simulink model "SG__MDL"  (R2022b)
settings: Solver=FixedStepAuto  StartTime=0.0  StopTime=Inf  FixedStep=5e-05  RelTol=1e-3  EnableMultiTasking=on
model workspace (MAT data in the model file):
  N_trig = Simulink.Parameter
  N_trig.Value = 32
  N_trig.Description = 'number of samples for triggered pulse for recording'
  N_trig.DataType = 'uint32'
  N_trig.Complexity = 'real'
  N_trig.Dimensions = [1 1]
  Sig = Simulink.Signal
  Sig.DataType = 'auto'
  Sig.Dimensions = -1
  Sig.DimensionsMode = 'auto'
  Sig.Complexity = 'auto'
  Sig.SampleTime = -1
  Sig.SamplingMode = 'auto'
  dtf_a = Simulink.Parameter
  dtf_a.Value = [1  1  1; 1  1  1]
  dtf_a.DataType = 'auto'
  dtf_a.Complexity = 'real'
  dtf_a.Dimensions = [2 3]
  dtf_b = Simulink.Parameter
  dtf_b.Value = [0.5  0.5  0.5; 0.5  0.5  0.5]
  dtf_b.DataType = 'auto'
  dtf_b.Complexity = 'real'
  dtf_b.Dimensions = [2 3]
  freq_0 = Simulink.Parameter
  freq_0.Value = 602
  freq_0.Description = 'tube fundamental resonance frequency
    | '
  freq_0.DataType = 'auto'
  freq_0.Complexity = 'real'
  freq_0.Dimensions = [1 1]
  i2u = Simulink.Parameter
  i2u.Value = 100
  i2u.Description = 'current to voltage conversion'
  i2u.DataType = 'auto'
  i2u.Complexity = 'real'
  i2u.Dimensions = [1 1]
  phi = Simulink.Parameter
  phi.Value = [0; 0]
  phi.DataType = 'auto'
  phi.Complexity = 'real'
  phi.Dimensions = [2 1]
  rec = Simulink.Parameter
  rec.Value = 0
  rec.DataType = 'boolean'
  rec.Complexity = 'real'
  rec.Dimensions = [1 1]
  rho = Simulink.Parameter
  rho.Value = [1; 1]
  rho.DataType = 'auto'
  rho.Complexity = 'real'
  rho.Dimensions = [2 1]
  sens_p = Simulink.Parameter
  sens_p.Value = [0; 0]
  sens_p.DataType = 'auto'
  sens_p.Complexity = 'real'
  sens_p.Dimensions = [2 1]
  src_gain = Simulink.Parameter
  src_gain.Value = 0.05
  src_gain.DataType = 'auto'
  src_gain.Complexity = 'real'
  src_gain.Dimensions = [1 1]
  theta = Simulink.Parameter
  theta.Value = [3.14159265359; 0]
  theta.DataType = 'auto'
  theta.Complexity = 'real'
  theta.Dimensions = [2 1]
  ts_ctr = Simulink.Parameter
  ts_ctr.Value = 5e-05
  ts_ctr.DataType = 'auto'
  ts_ctr.Complexity = 'real'
  ts_ctr.Dimensions = [1 1]
undefined symbols (not defined in the file or in its folder): gcbh, sps, sps_rtmsupport, t_s
libraries: simulink x3, speedgoatlib_IO135 x3, spsMeanLib x2, hdlsllib x2, slrealtimeloglib x1, dspsigops x1
settings Model: SimulationMode=external  ExtModeEnableFloating=off  DataflowThreadingImplementation=Pthreads  Creator=padlewsk  LastModifiedBy=padlewsk
settings SolverCC: ConcurrentTasks=on  AlgebraicLoopSolver=TrustRegion  PositivePriorityOrder=on  AutoInsertRateTranBlk=on
settings DataIOCC: SaveFormat=StructureWithTime
settings OptimizationCC: DefaultParameterBehavior=Inlined  GainParamInheritBuiltInType=on  UseFloatMulNetSlope=on  RollThreshold=9  EfficientFloat2IntCast=on  SimCompilerOptimization=on
settings DebuggingCC: ReadBeforeWriteMsg=DisableAll  WriteAfterWriteMsg=DisableAll  WriteAfterReadMsg=DisableAll  TasksWithSamePriorityMsg=none  UnconnectedInputMsg=warning  UnconnectedOutputMsg=warning  UnconnectedLineMsg=warning  ModelReferenceSymbolNameMessage=none
settings HardwareCC: ProdBitPerLong=64  ProdLongLongMode=on  ProdHWDeviceType=Intel->x86-64 (Linux 64)
settings ModelReferenceCC: UpdateModelReferenceTargets=IfOutOfDate  EnableRefExpFcnMdlSchedulingChecks=on
settings SFSimCC: SFSimEcho=off
settings RTWCC: Description=Simulink Real-Time  SystemTargetFile=slrealtime.tlc  TemplateMakefile=slrealtime_default_tmf  Toolchain=Simulink Real-Time Toolchain  BuildConfiguration=Faster Runs  CodeExecutionProfiling=on  TargetLang=C++
settings SimulinkRealTimeTargetCC: UseGCCFastMath=on

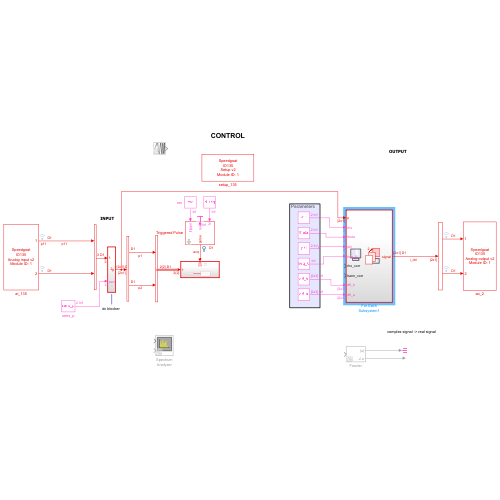
[thumbnail: Simulink's stored preview of the top-level diagram]
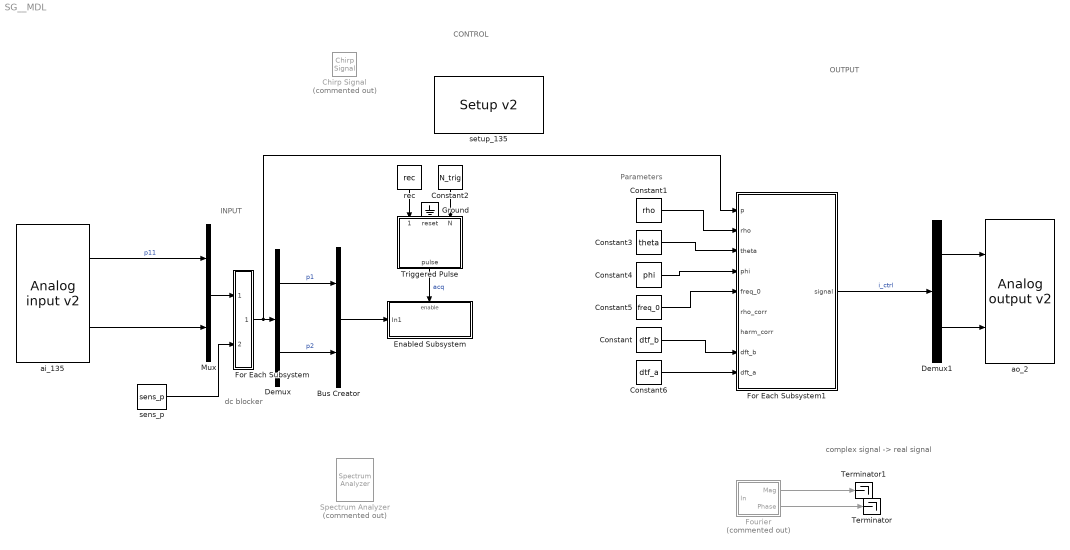
== system SG__MDL ==
  note: complex signal -> real signal
  note: dc blocker
  note: OUTPUT
  note: Parameters
  note: CONTROL
  note: INPUT
  Bus Creator : BusCreator  Inputs=2
  Chirp Signal : simulink/Sources/Chirp Signal  Commented=on  f1=10  T=10  f2=1500
  Constant : Constant  Value=dtf_b
  Constant1 : Constant  Value=rho
  Constant2 : Constant  Value=N_trig
  Constant3 : Constant  Value=theta
  Constant4 : Constant  Value=phi
  Constant5 : Constant  Value=freq_0
  Constant6 : Constant  Value=dtf_a
  Demux : Demux  Outputs=2
  Demux1 : Demux  Outputs=2
  Enabled Subsystem : Subsystem  TreatAsAtomicUnit=on
  For Each Subsystem : Subsystem  TreatAsAtomicUnit=on
  For Each Subsystem1 : Subsystem  TreatAsAtomicUnit=on
  Fourier : Subsystem  Commented=on  DialogController=POWERSYS.PowerSysDialog  LoadFcn=sps_rtmsupport('LoadFcn', gcbh);  StartFcn=sps_rtmsupport('StartFcn', gcbh);  StopFcn=sps_rtmsupport('StopFcn', gcbh);  mask(Fourier){Freq=freq_0, n=0, InInit=[0, 0], Ts=t_s}
      mask prompts: Freq "Fundamental frequency (Hz):"; n "Harmonic n (0=DC, 1=fundamental):"; InInit "Initial input [ Mag, Phase (degrees) ]:"; Ts "Sample time:"
      mask help:
      | Fourier analysis of the input signal over a running window of one cycle of the fundamental frequency.
      |
      | For the first cycle of simulation, the outputs are held  to the value specified in the Initial input parameter.
      mask init:
      | [WantBlockChoice,Ts,sps] = powericon('FourierInit',gcb,Freq,n,InInit,Ts);
      settings: LibrarySourceBlock=sps_lib/Sensors and Measurements/Fourier  CopyFcn=sps_rtmsupport('CopyFcn', gcbh);  DeleteFcn=sps_rtmsupport('DeleteFcn', gcbh);  UndoDeleteFcn=sps_rtmsupport('UndoDeleteFcn', gcbh);  ModelCloseFcn=sps_rtmsupport('ModelCloseFcn', gcbh);  PreSaveFcn=sps_rtmsupport('PreSaveFcn', gcbh);  PostSaveFcn=sps_rtmsupport('PostSaveFcn', gcbh);  NameChangeFcn=sps_rtmsupport('NameChangeFcn', gcbh);  PreCopyFcn=sps_rtmsupport('PreCopyFcn', gcbh);  OpenFcn=sps_rtmsupport('OpenFcn', gcbh, []);  CloseFcn=sps_rtmsupport('CloseFcn', gcbh);  PreDeleteFcn=sps_rtmsupport('PreDeleteFcn', gcbh);
      mask Help: helpview(psbhelp);
      mask Display:
      | port_label('output',1,'|u|')
      | port_label('output',2,'\angleu', 'texmode', 'on')
  Ground : Ground
  Mux : Mux  Inputs=2
  Spectrum Analyzer : SpectrumAnalyzer  Commented=on  NumInputPorts=2
  Terminator : Terminator
  Terminator1 : Terminator
  Triggered Pulse : Subsystem  mask(Triggered Pulse){}
      mask help: Generates a single pulse of N samples length
  ai_135 : speedgoatlib_IO135/Analog input v2   parModuleId=1  parSampleTime=-1  parPciSlot=-1  parAdcChannels=[1 2]  parAdcVoltageRange=[1 1 1 1]  parAdcOversamplRate=[1 1 1 1]  parAdcContSampling=0  parAdcDmaEnable=0  parAdcActiveDmaDevices=[1 1 1 1]  parAdcFrameSize=1
      settings: SourceProductName=Simulink Real-Time: Speedgoat I/O Blockset
  ao_2 : speedgoatlib_IO135/Analog output v2   parModuleId=1  parSampleTime=-1  parPciSlot=-1  parDacChannels=[1 2]  parDacVoltageRange=[4 4 4 4 4 4 4 4 4 4 4 4 4 4 4 4]  parDacInitValues=[0 0]  parDacReset=[1 1]  parDacSyncOut=1  parDacDmaEnable=0  parDacActiveDmaDevices=[1 1 1 1]  parDacDmaLatency=1  parDacFrameSize=1
      settings: SourceProductName=Simulink Real-Time: Speedgoat I/O Blockset
  rec : Constant  Value=rec
  sens_p : Constant  Value=sens_p
  setup_135 : speedgoatlib_IO135/Setup v2   parPciSlot=-1  parModuleId=1  parInterModuleSync=None  parConvClockBaseRate=20MHz  parConvClock1Divider=700  parConvClock2Divider=700  parFrameTriggerEnable=off  parFrameTriggerDivider=10  parConvClock1BaseRate=1  parConvClock2BaseRate=1  parFrameTriggerClock=1  parAdcChannels=[1:2]  parAdcRange1=+-5V  parAdcRange2=+-5V  parAdcRange3=+-5V  parAdcRange4=+-5V  parAdcVoltageRange=[1 1 1 1]  parAdcOversampling1=None  parAdcOversampling2=None  parAdcOversampling3=None  parAdcOversampling4=None  parAdcOversamplRate=[1 1 1 1]  parAdcAutoCorrection=on  parAdcContSampling=off  parAdcDmaEnable=off  parAdcDmaClock=Clock 1  parAdcFrameSize_=1  parAdcSampleTime_=-1  parAdcActiveDmaDevices=[1 1 1 1]  parAdcFrameTriggerEnable=0  parAdcFrameSize=1  parAdcSampleTime=3.5e-05  parDacChannels=[1:2]  parDacInitValues=zeros(1,2)  parDacReset=1  parDacRange1=+-5V  parDacRange2=+-5V  parDacRange3=+-5V  parDacRange4=+-5V  parDacRange5=+-5V  parDacRange6=+-5V  parDacRange7=+-5V  parDacRange8=+-5V  parDacRange9=+-5V  parDacRange10=+-5V  parDacRange11=+-5V  parDacRange12=+-5V  parDacRange13=+-5V  parDacRange14=+-5V  parDacRange15=+-5V  parDacRange16=+-5V  parDacVoltageRange=[4 4 4 4 4 4 4 4 4 4 4 4 4 4 4 4]  parDacAutoCorrection=on  parDacSyncOut=on  parDacDmaEnable=off  parDacDmaLatency=As small as possible  parDacDmaClock=Clock 1  parDacFrameSize_=1  parDacSampleTime_=-1  parDacActiveDmaDevices=[1 1 1 1]  parDacFrameTriggerEnable=0  parDacFrameSize=1  parDacSampleTime=3.5e-05  parDoChannels=[]  parDoInitValues=0  parDoReset=1  parDiChannels=[]  parDiDebounceEnable=off  parDiDebounceTime=0  parDiDebounceValue=0  parDioPullRefFront=Pull-up 3.3V  parDioPullRefRear=Floating
      settings: SourceProductName=Simulink Real-Time: Speedgoat I/O Blockset
  wires:
  ai_135/2 -> Mux/2
  ai_135/1 -> Mux/1  "p11"
  Mux/1 -> For Each Subsystem/1(In1)
  For Each Subsystem/1(p) -> For Each Subsystem1/1(p), Demux/1
  Bus Creator/1 -> Enabled Subsystem/1(In1)
  Demux/1 -> Bus Creator/1  "p1"
  Demux/2 -> Bus Creator/2  "p2"
  Triggered Pulse/1(pulse) -> Enabled Subsystem/Enable  "acq"
  Ground/1 -> Triggered Pulse/2(reset)
  rec/1 -> Triggered Pulse/1(trigger)
  Constant2/1 -> Triggered Pulse/3(N)
  Constant1/1 -> For Each Subsystem1/2(rho)
  Constant3/1 -> For Each Subsystem1/3(theta)
  Constant4/1 -> For Each Subsystem1/4(phi)
  Constant5/1 -> For Each Subsystem1/5(freq_0)
  Demux1/1 -> ao_2/1
  Demux1/2 -> ao_2/2
  Fourier/2(Phase) -> Terminator/1
  Fourier/1(Mag) -> Terminator1/1
  Constant6/1 -> For Each Subsystem1/9(dft_a)
  Constant/1 -> For Each Subsystem1/8(dft_b)
  For Each Subsystem1/1(signal) -> Demux1/1  "i_ctrl"
  sens_p/1 -> For Each Subsystem/2(sens_p)

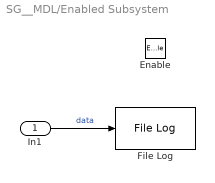
== system SG__MDL/Enabled Subsystem ==
  In1 : Inport
  Enable : EnablePort
  File Log : slrealtimeloglib/File Log  decimation=1  inputProcessing=Elements as channels (sample based)
  wires:
  In1/1 -> File Log/1  "data"

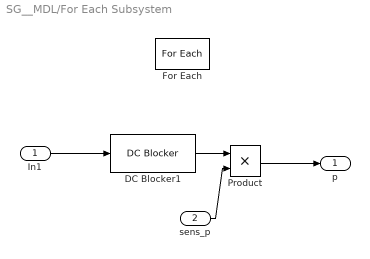
== system SG__MDL/For Each Subsystem ==
  In1 : Inport  Partition=on  PartitionDimension=1  PartitionWidth=1  PartitionOffset=0
  sens_p : Inport  Port=2  Partition=on  PartitionDimension=1  PartitionWidth=1  PartitionOffset=0
  DC Blocker1 : dspsigops/DC Blocker  Algorithm=IIR  NormalizedBandwidth=0.001  Length=50  Order=3  SimulateUsing=Code generation
      settings: LibrarySourceBlock=dsphdlsupportsigops/DC Blocker
  For Each : ForEach  DisableCoverage=on
  Product : Product
  p : Outport  ConcatenationDimension=1
  wires:
  In1/1 -> DC Blocker1/1
  DC Blocker1/1 -> Product/1
  Product/1 -> p/1
  sens_p/1 -> Product/2

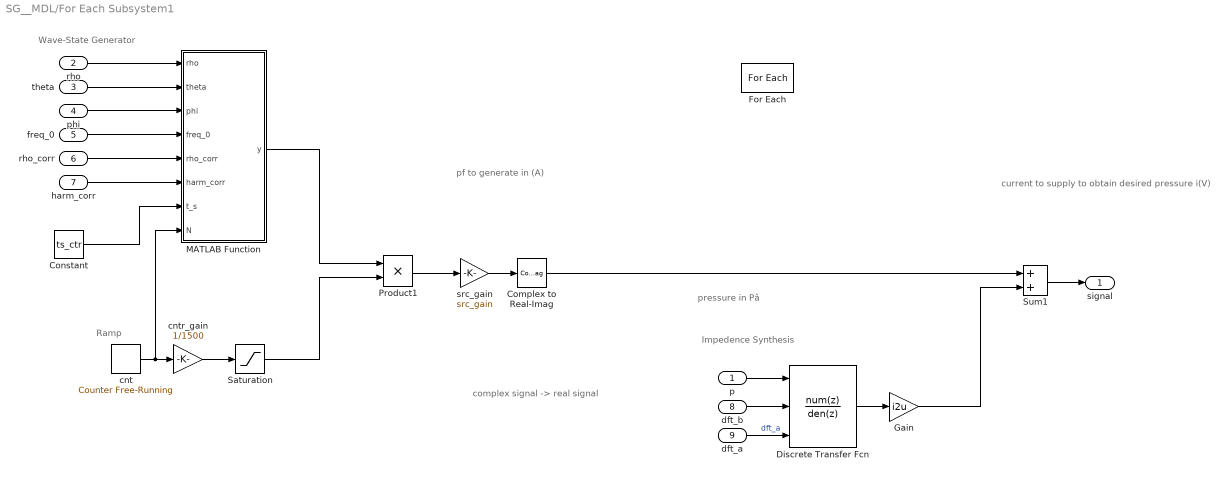
== system SG__MDL/For Each Subsystem1 ==
  note: pressure in Pâ
  note: pf to generate in (A)
  note: Wave-State Generator
  note: Impedence Synthesis
  note: Ramp
  note: complex signal -> real signal
  note: current to supply to obtain desired pressure i(V)
  p : Inport  Partition=on  PartitionDimension=1  PartitionWidth=1  PartitionOffset=0
  rho : Inport  Port=2  Partition=on  PartitionDimension=1  PartitionWidth=1  PartitionOffset=0
  theta : Inport  Port=3  Partition=on  PartitionDimension=1  PartitionWidth=1  PartitionOffset=0
  phi : Inport  Port=4  Partition=on  PartitionDimension=1  PartitionWidth=1  PartitionOffset=0
  freq_0 : Inport  Port=5
  rho_corr : Inport  Port=6
  harm_corr : Inport  Port=7
  dft_b : Inport  Port=8  Partition=on  PartitionDimension=1  PartitionWidth=1  PartitionOffset=0
  dft_a : Inport  Port=9  Partition=on  PartitionDimension=1  PartitionWidth=1  PartitionOffset=0
  Complex to Real-Imag : ComplexToRealImag  Output=Real
  Constant : Constant  Value=ts_ctr  SampleTime=-1
  Discrete Transfer Fcn : DiscreteTransferFcn  NumeratorSource=Input port  DenominatorSource=Input port  a0EqualsOne=on
      settings: InputPortMap=u0,p1,p3
  For Each : ForEach  DisableCoverage=on
  Gain : Gain  Gain=i2u
  MATLAB Function : MATLAB Function  TreatAsAtomicUnit=on
  Product1 : Product
  Saturation : Saturate  UpperLimit=1  LowerLimit=0
  Sum1 : Sum
  cnt : simulink/Sources/Counter Free-Running  NumBits=32  tsamp=-1
  cntr_gain : Gain  Gain=1/1500  ParamDataTypeStr=double
  src_gain : Gain  Gain=src_gain
  signal : Outport  OutputWhenDisabled=reset  InitialOutput=0  ConcatenationDimension=1  VectorParamsAs1DForOutWhenUnconnected=off
  wires:
  freq_0/1 -> MATLAB Function/4(freq_0)
  rho/1 -> MATLAB Function/1(rho)
  cnt/1 -> MATLAB Function/8(N), cntr_gain/1
  Product1/1 -> src_gain/1
  phi/1 -> MATLAB Function/3(phi)
  theta/1 -> MATLAB Function/2(theta)
  Saturation/1 -> Product1/2
  cntr_gain/1 -> Saturation/1
  Constant/1 -> MATLAB Function/7(t_s)
  MATLAB Function/1(y) -> Product1/1
  dft_b/1 -> Discrete Transfer Fcn/2
  dft_a/1 -> Discrete Transfer Fcn/3  "dft_a"
  src_gain/1 -> Complex to Real-Imag/1
  Discrete Transfer Fcn/1 -> Gain/1
  Gain/1 -> Sum1/2
  Sum1/1 -> signal/1
  p/1 -> Discrete Transfer Fcn/1
  Complex to Real-Imag/1 -> Sum1/1
  rho_corr/1 -> MATLAB Function/5(rho_corr)
  harm_corr/1 -> MATLAB Function/6(harm_corr)

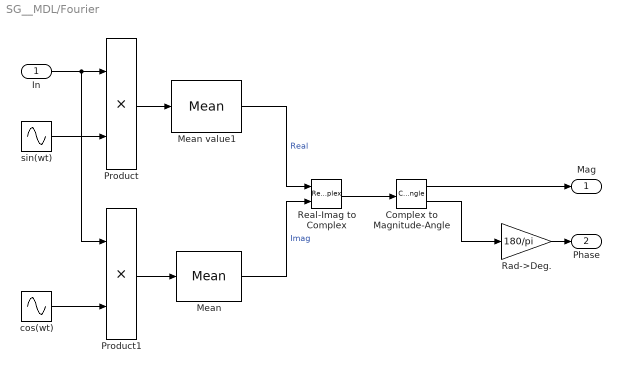
== system SG__MDL/Fourier ==
  In : Inport  SampleTime=Ts
  Complex to Magnitude-Angle : ComplexToMagnitudeAngle
  Mean : spsMeanLib/Mean  Freq=sps.Freq  Vinit=sps.Imag_Init  Ts=Ts
  Mean value1 : spsMeanLib/Mean  Freq=sps.Freq  Vinit=sps.Real_Init  Ts=Ts
  Product : Product  InputSameDT=on  SaturateOnIntegerOverflow=on  OutDataTypeStr=Inherit: Same as first input
  Product1 : Product  InputSameDT=on  SaturateOnIntegerOverflow=on  OutDataTypeStr=Inherit: Same as first input
  Rad->Deg. : Gain  Gain=180/pi  SaturateOnIntegerOverflow=on  OutDataTypeStr=Inherit: Same as input  ParamDataTypeStr=Inherit: Same as input
  Real-Imag to Complex : RealImagToComplex
  cos(wt) : Sin  Amplitude=sps.k  Frequency=2*pi*Freq*sps.n  Phase=pi/2  SampleTime=Ts
  sin(wt) : Sin  Amplitude=sps.k  Frequency=2*pi*Freq*sps.n  SampleTime=Ts
  Mag : Outport  SampleTime=Ts  VectorParamsAs1DForOutWhenUnconnected=off
  Phase : Outport  Port=2  SampleTime=Ts  VectorParamsAs1DForOutWhenUnconnected=off
  wires:
  In/1 -> Product/1, Product1/1
  sin(wt)/1 -> Product/2
  Product/1 -> Mean value1/1
  Mean value1/1 -> Real-Imag to Complex/1  "Real"
  Mean/1 -> Real-Imag to Complex/2  "Imag"
  Complex to Magnitude-Angle/1 -> Mag/1
  Rad->Deg./1 -> Phase/1
  Real-Imag to Complex/1 -> Complex to Magnitude-Angle/1
  Complex to Magnitude-Angle/2 -> Rad->Deg./1
  cos(wt)/1 -> Product1/2
  Product1/1 -> Mean/1

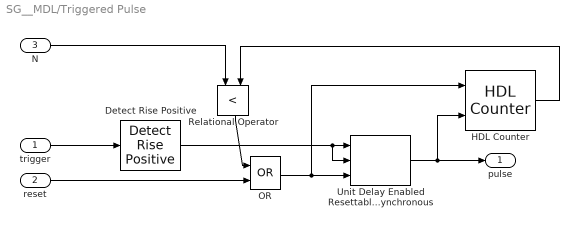
== system SG__MDL/Triggered Pulse ==
  trigger : Inport
  reset : Inport  Port=2
  N : Inport  Port=3
  Detect Rise Positive : simulink/Logic and Bit Operations/Detect Rise Positive  vinit=0  OutDataTypeStr=boolean
  HDL Counter : hdlsllib/Sources/HDL Counter  CountType=Free running  CountInit=1  CountStep=1  CountMax=25  CountFromType=Initial value  CountFrom=1  CountResetPort=on  CountLoadPort=off  CountEnbPort=on  CountDirPort=off  CountHitOutputPort=off  CountDataType=Unsigned  CountWordLen=32  CountFracLen=0  CountSampTime=1
  OR : Logic  Operator=OR  AllPortsSameDT=off  OutDataTypeStr=boolean
  Relational Operator : RelationalOperator  Operator=<  OutDataTypeStr=boolean  RndMeth=Simplest  InputSameDT=off
  Unit Delay Enabled Resettable Synchronous : hdlsllib/Discrete/Unit Delay Enabled Resettable Synchronous  InitialCondition=0.0  SampleTime=-1
  pulse : Outport  VectorParamsAs1DForOutWhenUnconnected=off
  wires:
  N/1 -> Relational Operator/1
  HDL Counter/1 -> Relational Operator/2
  Detect Rise Positive/1 -> Unit Delay Enabled Resettable Synchronous/2, Unit Delay Enabled Resettable Synchronous/1
  reset/1 -> OR/2
  Relational Operator/1 -> OR/1
  Unit Delay Enabled Resettable Synchronous/1 -> pulse/1, HDL Counter/2
  trigger/1 -> Detect Rise Positive/1
  OR/1 -> HDL Counter/1, Unit Delay Enabled Resettable Synchronous/3

== matlab function SG__MDL/For Each Subsystem1/MATLAB Function ==
  data: rho input; y output; theta input; phi input; freq_0 input; rho_corr input; harm_corr input; t_s input; N input
function y = fcn(rho,theta,phi,freq_0,rho_corr, harm_corr, t_s,N)
    omega_0 = 2*pi*freq_0;
    omega_1 = 2*omega_0;
    t = double(N)*t_s;
    psi = rho_corr*(rho*(cos(theta/2)*exp(-1i*omega_0*t) + harm_corr*sin(theta/2)*exp(1i*phi)*exp(-1i*omega_1*t)));
    y = psi;
end
